simulink model "model"  (R2018b)
settings: Solver=VariableStepAuto  StartTime=0.0  StopTime=10.0  RelTol=1e-3
libraries: slident x1, cstblocks x1
settings Model: Creator=Mark Sherstan  LastModifiedBy=Mark Sherstan

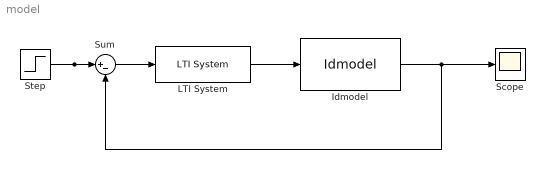
== system model ==
  Idmodel : slident/Models/Idmodel  sys=Plant1  IC=0  noi=off  seed=[]
      settings: SourceProductName=System Identification Toolbox  SourceProductBaseCode=ID
  LTI System : cstblocks/LTI System  sys=C  IC=[]
  Scope : Scope
  Step : Step  SampleTime=0
  Sum : Sum  Inputs=|+-
  wires:
  Step/1 -> Sum/1
  Sum/1 -> LTI System/1
  LTI System/1 -> Idmodel/1
  Idmodel/1 -> Sum/2, Scope/1
